simulink model "MPCFreq"  (R2021a)
settings: Solver=VariableStepAuto  StartTime=0.0  StopTime=0.3  FixedStep=1/150000  MaxStep=1e-6
libraries: spsMosfetLib x18, pid_lib x11, spsPermanentMagnetSynchronousMachineLib x3, simulink x3, spsCurrentMeasurementLib x3, spsDCVoltageSourceLib x3, spsThreePhaseVIMeasurementLib x3, spsabctodq0Lib x3, spsSVPWMGenerator2LevelLib x2, spsFirstOrderFilterLib x1, spsabctoAlphaBetaZeroLib x1, spsdq0toAlphaBetaZeroLib x1
(part 2 of 2)

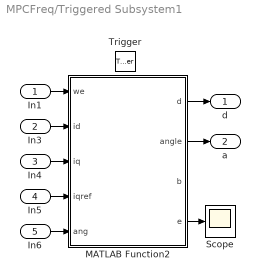
== system MPCFreq/Triggered Subsystem1 ==
  In1 : Inport
  In3 : Inport  Port=2
  In4 : Inport  Port=3
  In5 : Inport  Port=4
  In6 : Inport  Port=5
  Trigger : TriggerPort  VariantControl=Variant
  MATLAB Function2 : MATLAB Function  TreatAsAtomicUnit=on
  Scope : Scope
  d : Outport  VectorParamsAs1DForOutWhenUnconnected=off
  a : Outport  Port=2  VectorParamsAs1DForOutWhenUnconnected=off
  wires:
  MATLAB Function2/2(angle) -> a/1
  MATLAB Function2/1(d) -> d/1
  In6/1 -> MATLAB Function2/5(ang)
  In5/1 -> MATLAB Function2/4(iqref)
  In4/1 -> MATLAB Function2/3(iq)
  In3/1 -> MATLAB Function2/2(id)
  In1/1 -> MATLAB Function2/1(we)
  MATLAB Function2/4(e) -> Scope/1

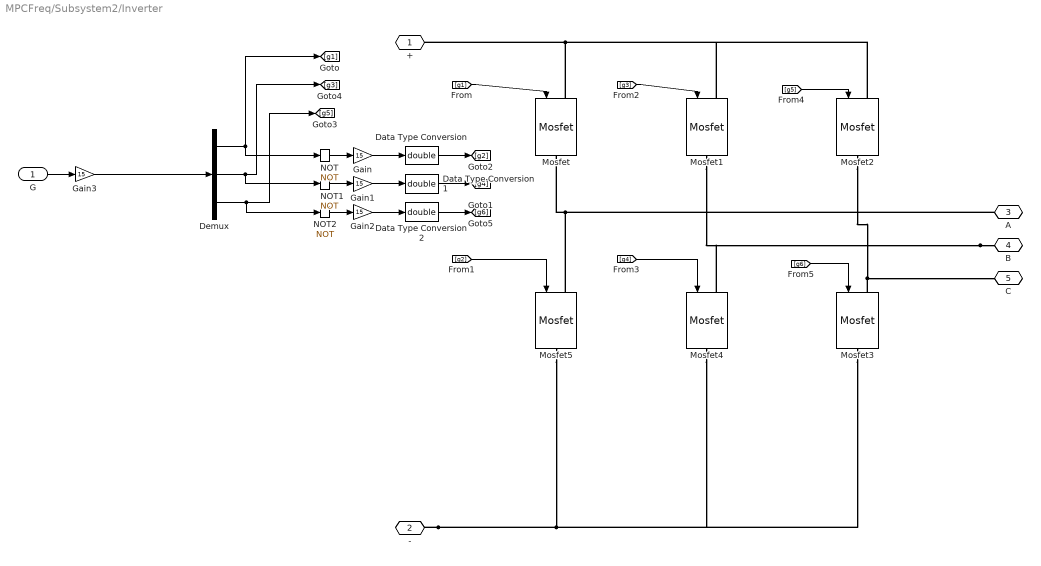
== system MPCFreq/Subsystem2/Inverter ==
  G : Inport
  Data Type Conversion : DataTypeConversion  OutDataTypeStr=double
  Data Type Conversion1 : DataTypeConversion  OutDataTypeStr=double
  Data Type Conversion2 : DataTypeConversion  OutDataTypeStr=double
  Demux : Demux  Outputs=3
  Gain{,1..3} (4 alike) : Gain  Gain=15
  Mosfet{,1..5} (6 alike) : spsMosfetLib/Mosfet  Ron=0.73  Lon=0  Rd=0.73  Vfd=1.15  IC=0  Rs=1e5  Cs=inf  Measurements=off
  NOT : Logic  Operator=NOT  IconShape=distinctive  AllPortsSameDT=off  OutDataTypeStr=boolean
  NOT1 : Logic  Operator=NOT  IconShape=distinctive  AllPortsSameDT=off  OutDataTypeStr=boolean
  NOT2 : Logic  Operator=NOT  IconShape=distinctive  AllPortsSameDT=off  OutDataTypeStr=boolean
  + : PMIOPort  Side=Left
  - : PMIOPort  Port=2  Side=Left
  A : PMIOPort  Port=3  Side=Right
  B : PMIOPort  Port=4  Side=Right
  C : PMIOPort  Port=5  Side=Right
  wires:
  [g2] -> Mosfet5/1
  [g6] -> Mosfet3/1
  [g1] -> Mosfet/1
  G/1 -> Gain3/1
  [g3] -> Mosfet1/1
  [g4] -> Mosfet4/1
  Demux/2 -> NOT1/1, [g3]
  Demux/3 -> NOT2/1, [g5]
  NOT/1 -> Gain/1
  NOT1/1 -> Gain1/1
  NOT2/1 -> Gain2/1
  Gain/1 -> Data Type Conversion/1
  Gain1/1 -> Data Type Conversion1/1
  Gain2/1 -> Data Type Conversion2/1
  Data Type Conversion/1 -> [g2]
  Data Type Conversion1/1 -> [g4]
  Data Type Conversion2/1 -> [g6]
  [g5] -> Mosfet2/1
  Gain3/1 -> Demux/1
  Demux/1 -> [g1], NOT/1
  connections:
  A/RConn1 -- Mosfet/RConn1 -- Mosfet5/LConn1
  B/RConn1 -- Mosfet4/LConn1 -- Mosfet1/RConn1
  Mosfet2/RConn1 -- C/RConn1 -- Mosfet3/LConn1
  Mosfet2/LConn1 -- Mosfet1/LConn1 -- Mosfet/LConn1 -- +/RConn1
  -/RConn1 -- Mosfet5/RConn1 -- Mosfet4/RConn1 -- Mosfet3/RConn1

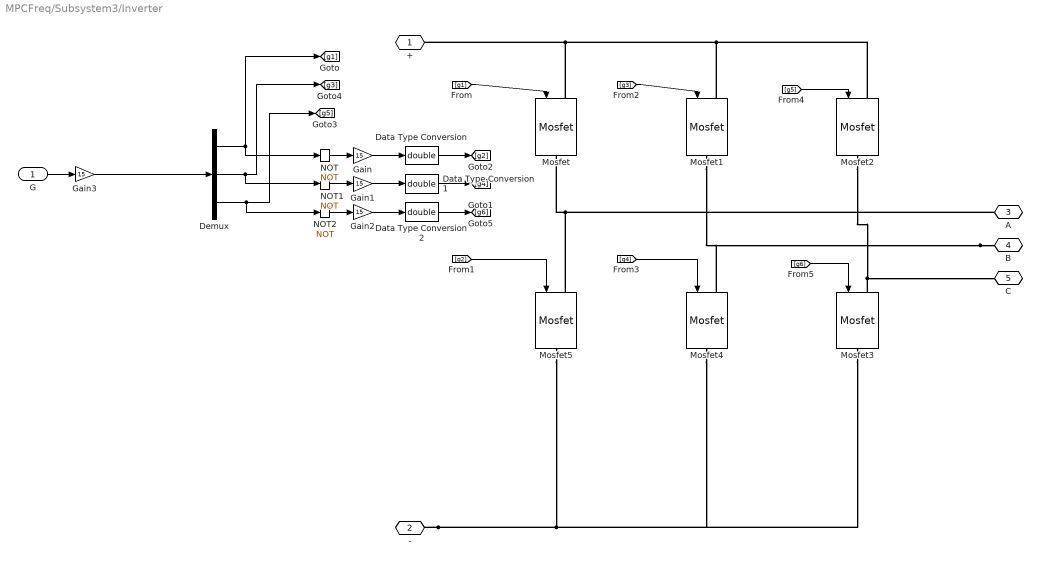
== system MPCFreq/Subsystem3/Inverter ==
  G : Inport
  Data Type Conversion : DataTypeConversion  OutDataTypeStr=double
  Data Type Conversion1 : DataTypeConversion  OutDataTypeStr=double
  Data Type Conversion2 : DataTypeConversion  OutDataTypeStr=double
  Demux : Demux  Outputs=3
  Gain{,1..3} (4 alike) : Gain  Gain=15
  Mosfet{,1..5} (6 alike) : spsMosfetLib/Mosfet  Ron=0.005  Lon=0  Rd=0.005  Vfd=1.15  IC=0  Rs=1e5  Cs=inf  Measurements=off
  NOT : Logic  Operator=NOT  IconShape=distinctive  AllPortsSameDT=off  OutDataTypeStr=boolean
  NOT1 : Logic  Operator=NOT  IconShape=distinctive  AllPortsSameDT=off  OutDataTypeStr=boolean
  NOT2 : Logic  Operator=NOT  IconShape=distinctive  AllPortsSameDT=off  OutDataTypeStr=boolean
  + : PMIOPort  Side=Left
  - : PMIOPort  Port=2  Side=Left
  A : PMIOPort  Port=3  Side=Right
  B : PMIOPort  Port=4  Side=Right
  C : PMIOPort  Port=5  Side=Right
  wires:
  [g2] -> Mosfet5/1
  [g6] -> Mosfet3/1
  [g1] -> Mosfet/1
  G/1 -> Gain3/1
  [g3] -> Mosfet1/1
  [g4] -> Mosfet4/1
  Demux/2 -> NOT1/1, [g3]
  Demux/3 -> NOT2/1, [g5]
  NOT/1 -> Gain/1
  NOT1/1 -> Gain1/1
  NOT2/1 -> Gain2/1
  Gain/1 -> Data Type Conversion/1
  Gain1/1 -> Data Type Conversion1/1
  Gain2/1 -> Data Type Conversion2/1
  Data Type Conversion/1 -> [g2]
  Data Type Conversion1/1 -> [g4]
  Data Type Conversion2/1 -> [g6]
  [g5] -> Mosfet2/1
  Gain3/1 -> Demux/1
  Demux/1 -> [g1], NOT/1
  connections:
  A/RConn1 -- Mosfet/RConn1 -- Mosfet5/LConn1
  B/RConn1 -- Mosfet4/LConn1 -- Mosfet1/RConn1
  Mosfet2/RConn1 -- C/RConn1 -- Mosfet3/LConn1
  Mosfet2/LConn1 -- Mosfet1/LConn1 -- Mosfet/LConn1 -- +/RConn1
  -/RConn1 -- Mosfet5/RConn1 -- Mosfet4/RConn1 -- Mosfet3/RConn1

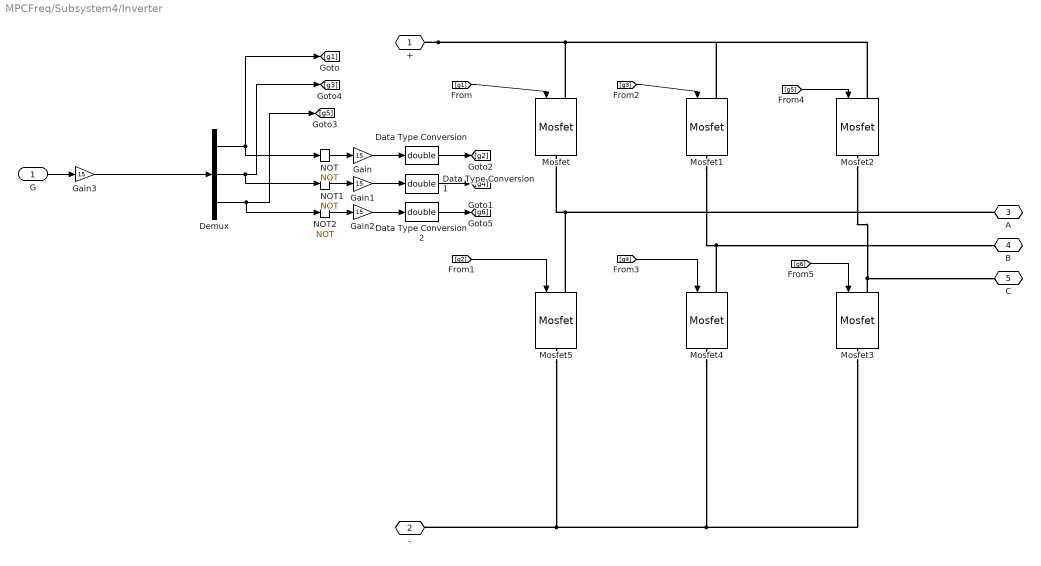
== system MPCFreq/Subsystem4/Inverter ==
  G : Inport
  Data Type Conversion : DataTypeConversion  OutDataTypeStr=double
  Data Type Conversion1 : DataTypeConversion  OutDataTypeStr=double
  Data Type Conversion2 : DataTypeConversion  OutDataTypeStr=double
  Demux : Demux  Outputs=3
  Gain{,1..3} (4 alike) : Gain  Gain=15
  Mosfet{,1..5} (6 alike) : spsMosfetLib/Mosfet  Ron=0.005  Lon=0  Rd=0.005  Vfd=1.15  IC=0  Rs=1e5  Cs=inf  Measurements=off
  NOT : Logic  Operator=NOT  IconShape=distinctive  AllPortsSameDT=off  OutDataTypeStr=boolean
  NOT1 : Logic  Operator=NOT  IconShape=distinctive  AllPortsSameDT=off  OutDataTypeStr=boolean
  NOT2 : Logic  Operator=NOT  IconShape=distinctive  AllPortsSameDT=off  OutDataTypeStr=boolean
  + : PMIOPort  Side=Left
  - : PMIOPort  Port=2  Side=Left
  A : PMIOPort  Port=3  Side=Right
  B : PMIOPort  Port=4  Side=Right
  C : PMIOPort  Port=5  Side=Right
  wires:
  Demux/1 -> NOT/1, [g1]
  Gain3/1 -> Demux/1
  [g5] -> Mosfet2/1
  Data Type Conversion2/1 -> [g6]
  Data Type Conversion1/1 -> [g4]
  Data Type Conversion/1 -> [g2]
  Gain2/1 -> Data Type Conversion2/1
  Gain1/1 -> Data Type Conversion1/1
  Gain/1 -> Data Type Conversion/1
  NOT2/1 -> Gain2/1
  NOT1/1 -> Gain1/1
  NOT/1 -> Gain/1
  Demux/3 -> [g5], NOT2/1
  Demux/2 -> [g3], NOT1/1
  [g4] -> Mosfet4/1
  [g3] -> Mosfet1/1
  G/1 -> Gain3/1
  [g1] -> Mosfet/1
  [g6] -> Mosfet3/1
  [g2] -> Mosfet5/1
  connections:
  Mosfet3/RConn1 -- Mosfet4/RConn1 -- Mosfet5/RConn1 -- -/RConn1
  +/RConn1 -- Mosfet/LConn1 -- Mosfet1/LConn1 -- Mosfet2/LConn1
  Mosfet3/LConn1 -- C/RConn1 -- Mosfet2/RConn1
  Mosfet1/RConn1 -- Mosfet4/LConn1 -- B/RConn1
  Mosfet5/LConn1 -- Mosfet/RConn1 -- A/RConn1

== matlab function MPCFreq/Triggered Subsystem1/MATLAB Function2 ==
  data: we input; id input; iq input; iqref input; ang input; d output; angle output; b output; e output
function [d,angle,b,e]  = MPC(we,id,iq,iqref,ang)

persistent oldState c sw sss;

if isempty(oldState)
    oldState = 1;
    psiq = 0;
    c  = 1;
    sw = 0;
    
    sss = [];
end
b = 0;
Ts = 1/20000;
Vdc = 12;
L = 0.0007;
R = 0.75;
psiPM = 0.00666;

p = 0.5;
q = 0.5;
r = 0.25;
s = 0.0;

states = [1 0    0 1    0 1;
         1 0    1 0    0 1;
         0 1    1 0    0 1;
         0 1    1 0    1 0;
         0 1    0 1    1 0;
         1 0    0 1    1 0;
         0 1    0 1    0 1;
         1 0    1 0    1 0];

y = states(1,:)';
cost = 10000000;

a = 1;

ang = ang - 2*pi*floor(ang/(2*pi));

ang = double(int16(ang*180/pi)*pi/180);

for i=1:6
    Sa=states(i,1);
    Sb=states(i,3);
    Sc=states(i,5);
    
    Va=(Vdc*(2*Sa-Sb-Sc))/3;
    Vb=(Vdc*(2*Sb-Sa-Sc))/3;
    Vc=(Vdc*(2*Sc-Sb-Sa))/3;
    
    vsd = round((3/2)*(sin(ang)*Va + sin(ang - (2*pi/3))*Vb + sin(ang + (2*pi/3))*Vc)*1000)/1000;
    vsq = round((3/2)*(cos(ang)*Va + cos(ang - (2*pi/3))*Vb + cos(ang + (2*pi/3))*Vc)*1000)/1000;
    
    vdx = round(-8*sin(ang - ((i-1)*pi/3))*1000)/1000;
    vqx = round(-8*sin(ang - (3*pi/2) + ((i-1)*pi/3))*1000)/1000;
    
    sss =[sss; vsd vdx];
    
    m = xor(states(i,[1,3,5]),states(oldState,[1,3,5]));
    
    m = length(find(m > 0));
    
    id_p = id;
    iq_p = iq;
    
    cTemp = 0;
    for x = 1:1
        xx = ((1-(R*Ts/L))*id_p)+(Ts*we*iq_p)+(vdx*Ts/L);
        yy = ((1-(R*Ts/L))*iq_p)-(Ts*we*id_p)-(psiPM*we*Ts/L)+(vqx*Ts/L);
    
        id_p = xx;
        iq_p = yy;

        cTemp = cTemp + (0 - id_p)^2 + 1.8*(iqref - iq_p)^2 + 0.00*m;
    end
    if(cTemp < cost)
       cost = cTemp;
       a = i;
    end
end

% if(abs(cost(a) - cost(oldState)) < 0.1)
%    a = oldState;
% end


if(a ~= oldState)
    c = c+1;
    
    if(a == 7 || a == 8)
       if(oldState == 1 || oldState == 3 || oldState == 5 || oldState == 8)
          a = 8; 
       elseif(oldState == 2 || oldState == 4 || oldState == 6 || oldState == 7)
           a = 7;
       end
    end
    
    oldState = a;
end
d=c;
sw = sw + 2*m;
b = a;
e = states(a,1);

angle = (a-1)*pi/3;
% angle = states(a,:);

== matlab function MPCFreq/Triggered Subsystem/MATLAB Function2 ==
  data: we input; id input; iq input; iqref input; ang input; d output; angle output; b output
function [d,angle,b]  = MPC(we,id,iq,iqref,ang)

persistent oldState c;

if isempty(oldState)
    oldState = 1;
    psiq = 0;
    c  = 1;
end
b = 0;
Ts = 1/20000;
Vdc = 12;
L = 0.0007;
R = 0.73+0.75;
psiPM = 0.00666;

p = 0.5;
q = 0.5;
r = 0.25;
s = 0.0;

states = [1 0    0 1    0 1;
         1 0    1 0    0 1;
         0 1    1 0    0 1;
         0 1    1 0    1 0;
         0 1    0 1    1 0;
         1 0    0 1    1 0;
         0 1    0 1    0 1;
         1 0    1 0    1 0];

y = states(1,:)';
cost = [];

for i=1:7
    Sa=states(i,1);
    Sb=states(i,3);
    Sc=states(i,5);
    
    Va=(Vdc*(2*Sa-Sb-Sc))/3;
    Vb=(Vdc*(2*Sb-Sa-Sc))/3;
    Vc=(Vdc*(2*Sc-Sb-Sa))/3;
    
    vsd = (2/3)*[sin(ang) sin(ang - (2*pi/3)) sin(ang + (2*pi/3))]*[Va Vb Vc]';
    vsq = (2/3)*[cos(ang) cos(ang - (2*pi/3)) cos(ang + (2*pi/3))]*[Va Vb Vc]';

    
    m = ~(states(i,:) == states(oldState,:));
    
    id_p = id;
    iq_p = iq;
    
    cTemp = 0;
    for x = 1:1
        xx = ((1-(R*Ts/L))*id_p)+(Ts*we*iq_p)+(vsd*Ts/L);
        yy = ((1-(R*Ts/L))*iq_p)-(Ts*we*id_p)-(psiPM*we*Ts/L)+(vsq*Ts/L);
    
        id_p = xx;
        iq_p = yy;
        
        ia = cos(ang)*id_p - sin(ang)*iq_p;
        ib = cos(ang - (2*pi/3))*id_p - sin(ang - (2*pi/3))*iq_p;
        ic = cos(ang + (2*pi/3))*id_p - sin(ang + (2*pi/3))*iq_p;
% 
%         if abs(iq_p) > 3
%             cTemp = cTemp + 1000*abs(3 - sqrt(id_p^2 + iq_p^2));
%         end
        
        cTemp = cTemp + (0 - id_p)^2 + 1.8*(iqref - iq_p)^2;
    end
    

    cost = [cost  cTemp];
end

a = find(cost == min(cost));
a = a(end);

% if(abs(cost(a) - cost(oldState)) < 0.1)
%    a = oldState;
% end


if(a ~= oldState)
    c = c+1;
    
    if(a == 7 || a == 8)
       if(oldState == 1 || oldState == 3 || oldState == 5 || oldState == 8)
          a = 8; 
       elseif(oldState == 2 || oldState == 4 || oldState == 6 || oldState == 7)
           a = 7;
       end
    end
    
    oldState = a;
end
d=c;

b = a;

% angle = (a-1)*pi/3;
angle = states(a,:);
